simulink model "ee463_project_simulation_updated"  (R2023b)
settings: Solver=VariableStepAuto  StartTime=0.0  StopTime=0.04  RelTol=1e-3
undefined symbols (not defined in the file or in its folder): Acid, Lead
libraries: spsDiodeLib x8, spsVoltageMeasurementLib x7, spsCurrentMeasurementLib x4, spsSeriesRLCBranchLib x4, spsACVoltageSourceLib x3, spsBatteryLib x2, spsMeanLib x1, spsMosfetLib x1, spsRMSLib x1, sps_lib x1
settings Model: Creator=Emir  LastModifiedBy=Emir

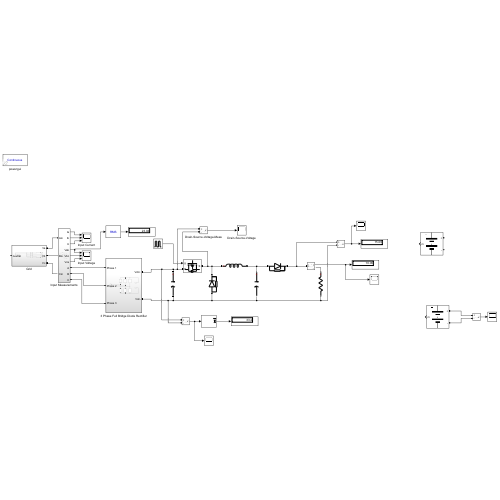
[thumbnail: Simulink's stored preview of the top-level diagram]
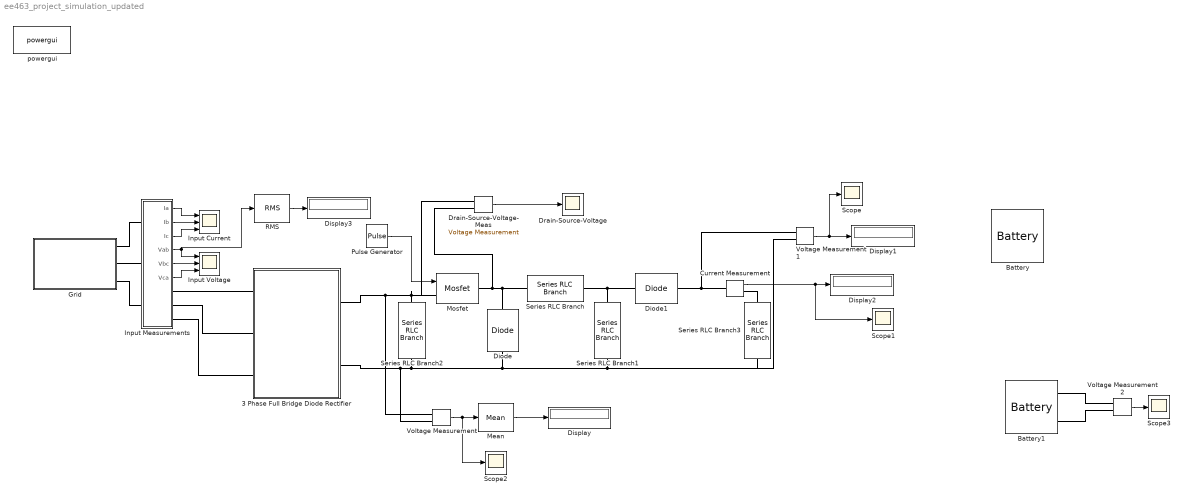
== system ee463_project_simulation_updated ==
  3 Phase Full Bridge Diode Rectifier : Subsystem
  Battery : spsBatteryLib/Battery  BatType=Lead-Acid  ShowTempParam=off  ThermalPreset=no  ShowAgeParam=off  NomV=12  NomQ=100  SOC=80  Batt_Tr=30  PresetModel=on  MaxQ=104.1667  MinV=9  FullV=13.0658  Dis_rate=20  R=0.0012  Normal_OP=31.0278  expZone="[12.2171     0.333333]"  current=[6.5 13 32.5]  Units=Time  Tci=20  NomT=20  T2=-30  MaxQ2=4.8  FullV2=7.1  Normal_OP2=5.655  expZone2="[6.58           1]"  Rca=0.6  ti=2000  Dp=0  Neq0=0  Tsim=1e6  Ta1=25  Qeol=5.4*0.9  Reol=0.013333*1.2  Char_age=[2.3478, 3]  Dis_age=[2.3478, 10]  N1=1500  N2=10500  N3=1000  N4=1400  Ta2=45  N5=950
  Battery1 : spsBatteryLib/Battery  BatType=Lead-Acid  ShowTempParam=off  ThermalPreset=no  ShowAgeParam=off  NomV=12  NomQ=100  SOC=0  Batt_Tr=30  PresetModel=on  MaxQ=104.1667  MinV=9  FullV=13.0658  Dis_rate=20  R=0.0012  Normal_OP=31.0278  expZone="[12.2171     0.333333]"  current=[6.5 13 32.5]  Units=Time  Tci=20  NomT=20  T2=-30  MaxQ2=4.8  FullV2=7.1  Normal_OP2=5.655  expZone2="[6.58           1]"  Rca=0.6  ti=2000  Dp=0  Neq0=0  Tsim=1e6  Ta1=25  Qeol=5.4*0.9  Reol=0.013333*1.2  Char_age=[2.3478, 3]  Dis_age=[2.3478, 10]  N1=1500  N2=10500  N3=1000  N4=1400  Ta2=45  N5=950
  Current Measurement : spsCurrentMeasurementLib/Current Measurement  PhasorSimulation=off  OutputType=Complex  PSBequivalent=0
  Diode : spsDiodeLib/Diode  Ron=0.001  Lon=0  Vf=0.8  IC=0  UseSnubber=0  Rs=500  Cs=250e-9  Measurements=off
  Diode1 : spsDiodeLib/Diode  Ron=0.001  Lon=0  Vf=0.8  IC=0  UseSnubber=0  Rs=500  Cs=250e-9  Measurements=off
  Display{,1..3} (4 alike) : Display
  Drain-Source-Voltage : Scope
  Drain-Source-Voltage-Meas : spsVoltageMeasurementLib/Voltage Measurement  PhasorSimulation=off  OutputType=Complex  PSBequivalent=0
  Grid : Subsystem
  Input Current : Scope  NumInputPorts=3
  Input Measurements : Subsystem
  Input Voltage : Scope  NumInputPorts=3
  Mean : spsMeanLib/Mean  Freq=60  Vinit=0  Ts=0
  Mosfet : spsMosfetLib/Mosfet  Ron=0.1  Lon=0  Rd=0.01  Vfd=0  IC=0  Rs=1e5  Cs=inf  Measurements=off
  Pulse Generator : DiscretePulseGenerator  PulseType=Time based  Period=1e-5  PulseWidth=50
  RMS : spsRMSLib/RMS  TrueRMS=on  Freq=60  RMSInit=120  Ts=0
  Scope{,1..3} (4 alike) : Scope
  Series RLC Branch : spsSeriesRLCBranchLib/Series RLC Branch  LConnTagsString=__new0  RConnTagsString=__new0  BranchType=L  Resistance=1  Inductance=100e-6  SetiL0=off  InitialCurrent=0  Capacitance=1e-6  Setx0=off  InitialVoltage=0  Measurements=None
  Series RLC Branch1 : spsSeriesRLCBranchLib/Series RLC Branch  LConnTagsString=__new0  RConnTagsString=__new0  BranchType=C  Resistance=100  Inductance=1e-3  SetiL0=off  InitialCurrent=0  Capacitance=4.7e-6  Setx0=off  InitialVoltage=0  Measurements=None
  Series RLC Branch2 : spsSeriesRLCBranchLib/Series RLC Branch  LConnTagsString=__new0  RConnTagsString=__new0  BranchType=C  Resistance=100  Inductance=1e-3  SetiL0=off  InitialCurrent=0  Capacitance=10000e-6  Setx0=off  InitialVoltage=0  Measurements=None
  Series RLC Branch3 : spsSeriesRLCBranchLib/Series RLC Branch  LConnTagsString=__new0  RConnTagsString=__new0  BranchType=R  Resistance=1.5  Inductance=1e-3  SetiL0=off  InitialCurrent=0  Capacitance=1000e-6  Setx0=off  InitialVoltage=0  Measurements=None
  Voltage Measurement : spsVoltageMeasurementLib/Voltage Measurement  PhasorSimulation=off  OutputType=Complex  PSBequivalent=0
  Voltage Measurement1 : spsVoltageMeasurementLib/Voltage Measurement  PhasorSimulation=off  OutputType=Complex  PSBequivalent=0
  Voltage Measurement2 : spsVoltageMeasurementLib/Voltage Measurement  PhasorSimulation=off  OutputType=Complex  PSBequivalent=0
  powergui : sps_lib/powergui  Priority=1  SimulationMode=Continuous  SampleTime=50e-6  frequency=60  Iterations=50  frequencyindice=0  Pbase=100e6  ErrMax=1e-4  UnitsV=kV  UnitsW=MW  buscounter=0  FunctionMessages=off  echomessages=off  EnableUseOfTLC=off  CurrentSourceSwitches=off  DisableSnubberDevices=off  DisableRonSwitches=off  DisableVfSwitches=off  DisplayEquations=off  AutomaticDiscreteSolvers=off  SolverType=Tustin/Backward Euler (TBE)  Interpol=off  ExternalGateDelay=off  methode=off  Ts=100  x0status=blocks  SPID=on  SwTol=0  HookPort=off  NonlinearTolerance=1e-4  nMaxIteration=100  ContinueOnMaxIteration=off  RestoreLinks=warning  ResistiveCurrentMeasurement=off  Frange=[0:2:500]  Ylog=off  Xlog=on  ShowGrid=off  save=off  variable=ZData  structure=0  ZoomFFT=off  StartTime=0.0  cycles=1  DisplayStyle=1  fundamental=60  FreqAxis=off  MaxFrequency=1000  frequencyindicesteady=1  RmsSteady=1  display=off
  wires:
  Voltage Measurement/1 -> Scope2/1, Mean/1
  Mean/1 -> Display/1
  Voltage Measurement1/1 -> Scope/1, Display1/1
  Current Measurement/1 -> Scope1/1, Display2/1
  Pulse Generator/1 -> Mosfet/1
  Drain-Source-Voltage-Meas/1 -> Drain-Source-Voltage/1
  Input Measurements/1(Ia) -> Input Current/1
  Input Measurements/4(Vab) -> RMS/1, Input Voltage/1
  Input Measurements/2(Ib) -> Input Current/2
  Input Measurements/5(Vbc) -> Input Voltage/2
  Input Measurements/3(Ic) -> Input Current/3
  Input Measurements/6(Vca) -> Input Voltage/3
  RMS/1 -> Display3/1
  Voltage Measurement2/1 -> Scope3/1
  connections:
  Series RLC Branch3/RConn1 -- Voltage Measurement1/LConn2 -- Series RLC Branch1/RConn1 -- Diode/LConn1 -- Voltage Measurement/LConn2 -- 3 Phase Full Bridge Diode Rectifier/RConn2 -- Series RLC Branch2/RConn1
  Drain-Source-Voltage-Meas/LConn1 -- Mosfet/LConn1 -- Voltage Measurement/LConn1 -- 3 Phase Full Bridge Diode Rectifier/RConn1 -- Series RLC Branch2/LConn1
  Mosfet/RConn1 -- Drain-Source-Voltage-Meas/LConn2 -- Diode/RConn1 -- Series RLC Branch/LConn1
  Series RLC Branch1/LConn1 -- Diode1/LConn1 -- Series RLC Branch/RConn1
  Voltage Measurement1/LConn1 -- Current Measurement/LConn1 -- Diode1/RConn1
  Input Measurements/RConn1 -- 3 Phase Full Bridge Diode Rectifier/LConn1
  Grid/RConn1 -- Input Measurements/LConn1
  Input Measurements/LConn2 -- Grid/RConn2
  Input Measurements/RConn2 -- 3 Phase Full Bridge Diode Rectifier/LConn2
  Grid/RConn3 -- Input Measurements/LConn3
  Input Measurements/RConn3 -- 3 Phase Full Bridge Diode Rectifier/LConn3
  Battery1/LConn1 -- Voltage Measurement2/LConn1
  Battery1/LConn2 -- Voltage Measurement2/LConn2
  Series RLC Branch3/LConn1 -- Current Measurement/RConn1

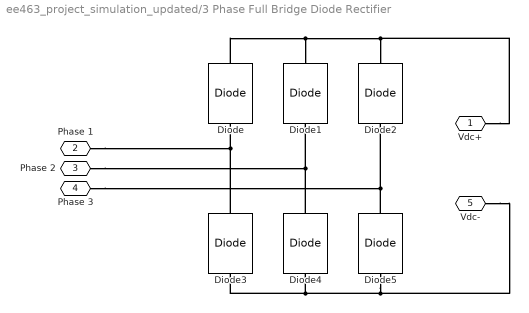
== system ee463_project_simulation_updated/3 Phase Full Bridge Diode Rectifier ==
  Diode{,1..5} (6 alike) : spsDiodeLib/Diode  Ron=0.001  Lon=0  Vf=0.8  IC=0  UseSnubber=0  Rs=500  Cs=250e-9  Measurements=off
  Vdc+ : PMIOPort  Side=Right
  Phase 1 : PMIOPort  Port=2  Side=Left
  Phase 2 : PMIOPort  Port=3  Side=Left
  Phase 3 : PMIOPort  Port=4  Side=Left
  Vdc- : PMIOPort  Port=5  Side=Right
  connections:
  Diode4/RConn1 -- Phase 2/RConn1 -- Diode1/LConn1
  Diode5/RConn1 -- Phase 3/RConn1 -- Diode2/LConn1
  Diode/RConn1 -- Diode1/RConn1 -- Vdc+/RConn1 -- Diode2/RConn1
  Diode3/RConn1 -- Phase 1/RConn1 -- Diode/LConn1
  Diode5/LConn1 -- Vdc-/RConn1 -- Diode4/LConn1 -- Diode3/LConn1

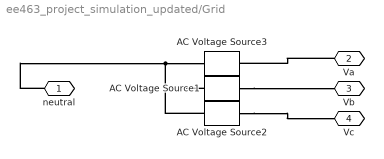
== system ee463_project_simulation_updated/Grid ==
  AC Voltage Source1 : spsACVoltageSourceLib/AC Voltage Source  Amplitude=20.41  Phase=-120  Frequency=50  SampleTime=0  Measurements=None  BusType=swing  Pref=10e3  Qref=0  Qmin=-inf  Qmax=+inf
  AC Voltage Source2 : spsACVoltageSourceLib/AC Voltage Source  Amplitude=20.41  Phase=120  Frequency=50  SampleTime=0  Measurements=None  BusType=swing  Pref=10e3  Qref=0  Qmin=-inf  Qmax=+inf
  AC Voltage Source3 : spsACVoltageSourceLib/AC Voltage Source  Amplitude=20.41  Phase=0  Frequency=50  SampleTime=0  Measurements=None  BusType=swing  Pref=10e3  Qref=0  Qmin=-inf  Qmax=+inf
  neutral : PMIOPort  Side=Left
  Va : PMIOPort  Port=2  Side=Right
  Vb : PMIOPort  Port=3  Side=Right
  Vc : PMIOPort  Port=4  Side=Right
  connections:
  AC Voltage Source1/RConn1 -- Vb/RConn1
  Va/RConn1 -- AC Voltage Source3/RConn1
  AC Voltage Source2/RConn1 -- Vc/RConn1
  neutral/RConn1 -- AC Voltage Source2/LConn1 -- AC Voltage Source1/LConn1 -- AC Voltage Source3/LConn1

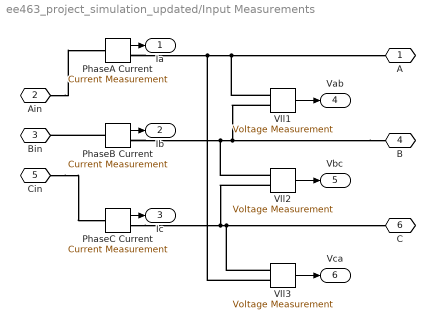
== system ee463_project_simulation_updated/Input Measurements ==
  PhaseA Current : spsCurrentMeasurementLib/Current Measurement  PhasorSimulation=off  OutputType=Complex  PSBequivalent=0
  PhaseB Current : spsCurrentMeasurementLib/Current Measurement  PhasorSimulation=off  OutputType=Complex  PSBequivalent=0
  PhaseC Current : spsCurrentMeasurementLib/Current Measurement  PhasorSimulation=off  OutputType=Complex  PSBequivalent=0
  Vll1 : spsVoltageMeasurementLib/Voltage Measurement  PhasorSimulation=off  OutputType=Complex  PSBequivalent=0
  Vll2 : spsVoltageMeasurementLib/Voltage Measurement  PhasorSimulation=off  OutputType=Complex  PSBequivalent=0
  Vll3 : spsVoltageMeasurementLib/Voltage Measurement  PhasorSimulation=off  OutputType=Complex  PSBequivalent=0
  A : PMIOPort  Side=Right
  Ain : PMIOPort  Port=2  Side=Left
  Bin : PMIOPort  Port=3  Side=Left
  B : PMIOPort  Port=4  Side=Right
  Cin : PMIOPort  Port=5  Side=Left
  C : PMIOPort  Port=6  Side=Right
  Ia : Outport
  Ib : Outport  Port=2
  Ic : Outport  Port=3
  Vab : Outport  Port=4
  Vbc : Outport  Port=5
  Vca : Outport  Port=6
  wires:
  PhaseC Current/1 -> Ic/1
  Vll3/1 -> Vca/1
  PhaseA Current/1 -> Ia/1
  PhaseB Current/1 -> Ib/1
  Vll1/1 -> Vab/1
  Vll2/1 -> Vbc/1
  connections:
  PhaseB Current/RConn1 -- Vll2/LConn1 -- Vll1/LConn2 -- B/RConn1
  PhaseA Current/RConn1 -- Vll3/LConn2 -- A/RConn1 -- Vll1/LConn1
  Cin/RConn1 -- PhaseC Current/LConn1
  Ain/RConn1 -- PhaseA Current/LConn1
  PhaseC Current/RConn1 -- C/RConn1 -- Vll3/LConn1 -- Vll2/LConn2
  PhaseB Current/LConn1 -- Bin/RConn1
